simulink model "ProyectoAutomatasSimulink_jona2015a"  (R2015a)
settings: Solver=ode45  SolverMode=SingleTasking  StartTime=0.0  StopTime=100  RelTol=1e-3
undefined symbols (not defined in the file or in its folder): bh, bt, bw, g, Jh, Kw, Mh, ml, ml0, mlempty, mlfull, Mt, rc, Rd, rh, Rw, Thmax, Ttmax, yt0
settings Model: Creator=Maxi Garcia  LastModifiedBy=yellow submarine
settings DataIOCC: SignalLoggingSaveFormat=ModelDataLogs
settings OptimizationCC: BlockReduction=off  BooleanDataType=off
settings DebuggingCC: SaveWithParameterizedLinksMsg=none  UnderspecifiedInitializationDetection=Classic  MergeDetectMultiDrivingBlocksExec=none  SignalResolutionControl=TryResolveAllWithWarning  MultiTaskDSMMsg=warning  MultiTaskCondExecSysMsg=none
settings HardwareCC: TargetUnknown=on

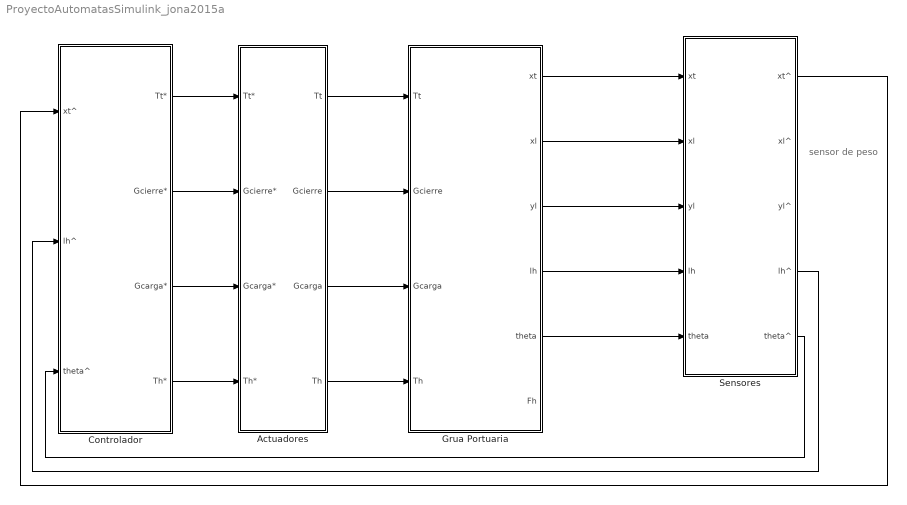
== system ProyectoAutomatasSimulink_jona2015a ==
  note: sensor de peso
  Actuadores : Subsystem
  Controlador : Subsystem
  Grua Portuaria : Subsystem
  Sensores : Subsystem
  wires:
  Grua Portuaria/1(xt) -> Sensores/1(xt)
  Grua Portuaria/2(xl) -> Sensores/2(xl)
  Grua Portuaria/3(yl) -> Sensores/3(yl)
  Grua Portuaria/4(lh) -> Sensores/4(lh)
  Grua Portuaria/5(theta) -> Sensores/5(theta)
  Actuadores/1(Tt) -> Grua Portuaria/1(Tt)
  Actuadores/2(Gcierre) -> Grua Portuaria/2(Gcierre)
  Actuadores/3(Gcarga) -> Grua Portuaria/3(Gcarga)
  Actuadores/4(Th) -> Grua Portuaria/4(Th)
  Controlador/1(Tt*) -> Actuadores/1(Tt*)
  Controlador/4(Th*) -> Actuadores/4(Th*)
  Controlador/2(Gcierre*) -> Actuadores/2(Gcierre*)
  Controlador/3(Gcarga*) -> Actuadores/3(Gcarga*)
  Sensores/5(theta^) -> Controlador/3(theta^)
  Sensores/4(lh^) -> Controlador/2(lh^)
  Sensores/1(xt^) -> Controlador/1(xt^)

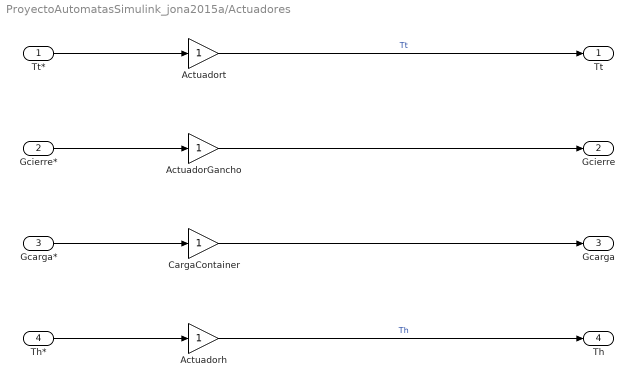
== system ProyectoAutomatasSimulink_jona2015a/Actuadores ==
  Tt* : Inport
  Gcierre* : Inport  Port=2
  Gcarga* : Inport  Port=3
  Th* : Inport  Port=4
  ActuadorGancho : Gain
  Actuadorh : Gain
  Actuadort : Gain
  CargaContainer : Gain
  Tt : Outport
  Gcierre : Outport  Port=2
  Gcarga : Outport  Port=3
  Th : Outport  Port=4
  wires:
  Th*/1 -> Actuadorh/1
  Actuadort/1 -> Tt/1  "Tt"
  Tt*/1 -> Actuadort/1
  ActuadorGancho/1 -> Gcierre/1
  CargaContainer/1 -> Gcarga/1
  Actuadorh/1 -> Th/1  "Th"
  Gcierre*/1 -> ActuadorGancho/1
  Gcarga*/1 -> CargaContainer/1

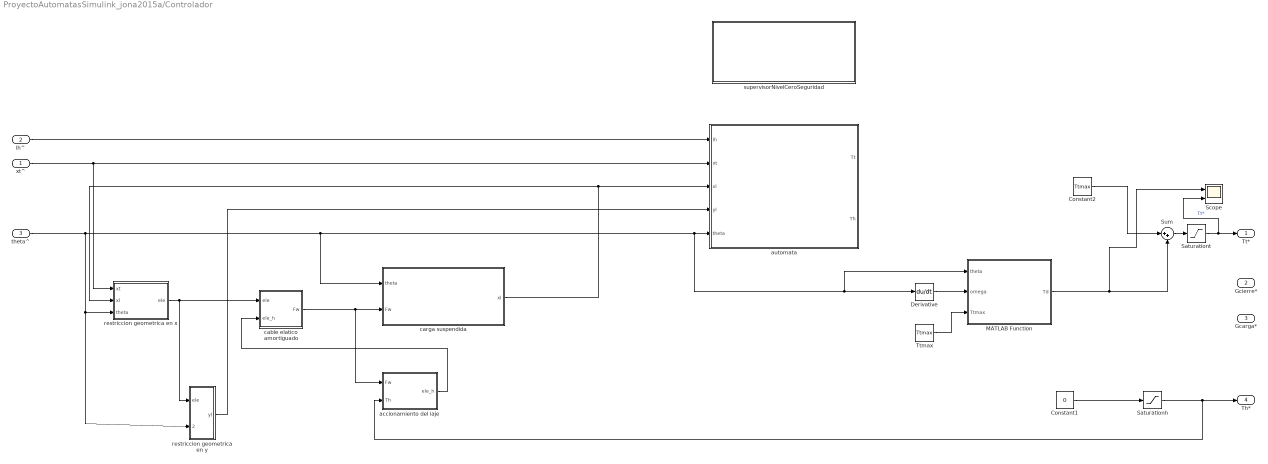
== system ProyectoAutomatasSimulink_jona2015a/Controlador ==
  xt^ : Inport
  lh^ : Inport  Port=2
  theta^ : Inport  Port=3
  Constant1 : Constant  Value=0
  Constant2 : Constant  Value=Ttmax
  Derivative : Derivative
  MATLAB Function : MATLAB Function  TreatAsAtomicUnit=on
      settings: PermitHierarchicalResolution=ParametersOnly
  Saturationh : Saturate  UpperLimit=Thmax  LowerLimit=-Ttmax
  Saturationt : Saturate  UpperLimit=Ttmax  LowerLimit=-Ttmax
  Scope : Scope  NumInputPorts=2
      settings: TimeRange=auto  MaxDataPoints=5000  SaveToWorkspace=off  YMin=-600000~-400000  YMax=800000~400000  SampleTime=-1  DataFormat=Array
  Sum : Sum  Inputs=|++
  Ttmax : Constant  Value=Ttmax
  accionamiento del iaje : Subsystem
  automata : Stateflow chart  TreatAsAtomicUnit=on
      settings: PermitHierarchicalResolution=ParametersOnly
  cable elatico amortiguado : Subsystem
  carga suspendida : Subsystem
  restriccion geometrica en x : Subsystem
  restriccion geometrica en y : Subsystem
  supervisorNivelCeroSeguridad : Stateflow chart  TreatAsAtomicUnit=on
      settings: PermitHierarchicalResolution=ParametersOnly
  Tt* : Outport
  Gcierre* : Outport  Port=2
  Gcarga* : Outport  Port=3
  Th* : Outport  Port=4
  wires:
  Saturationt/1 -> Scope/2, Tt*/1  "Tt*"
  MATLAB Function/1(Td) -> Sum/2, Scope/1
  Constant1/1 -> Saturationh/1
  theta^/1 -> restriccion geometrica en y/2(theta), restriccion geometrica en x/3(theta), carga suspendida/1(theta), Derivative/1, MATLAB Function/1(theta), automata/5(theta)
  Derivative/1 -> MATLAB Function/2(omega)
  Ttmax/1 -> MATLAB Function/3(Ttmax)
  Sum/1 -> Saturationt/1
  Constant2/1 -> Sum/1
  xt^/1 -> restriccion geometrica en x/1(xt), automata/2(xt)
  lh^/1 -> automata/1(lh)
  carga suspendida/1(xl) -> restriccion geometrica en x/2(xl), automata/3(xl)
  cable elatico amortiguado/1(Fw) -> accionamiento del iaje/1(Fw), carga suspendida/2(Fw)
  restriccion geometrica en x/1(ele) -> restriccion geometrica en y/1(ele), cable elatico amortiguado/1(ele)
  Saturationh/1 -> accionamiento del iaje/2(Th), Th*/1
  accionamiento del iaje/1(ele_h) -> cable elatico amortiguado/2(ele_h)
  restriccion geometrica en y/1(yl) -> automata/4(yl)

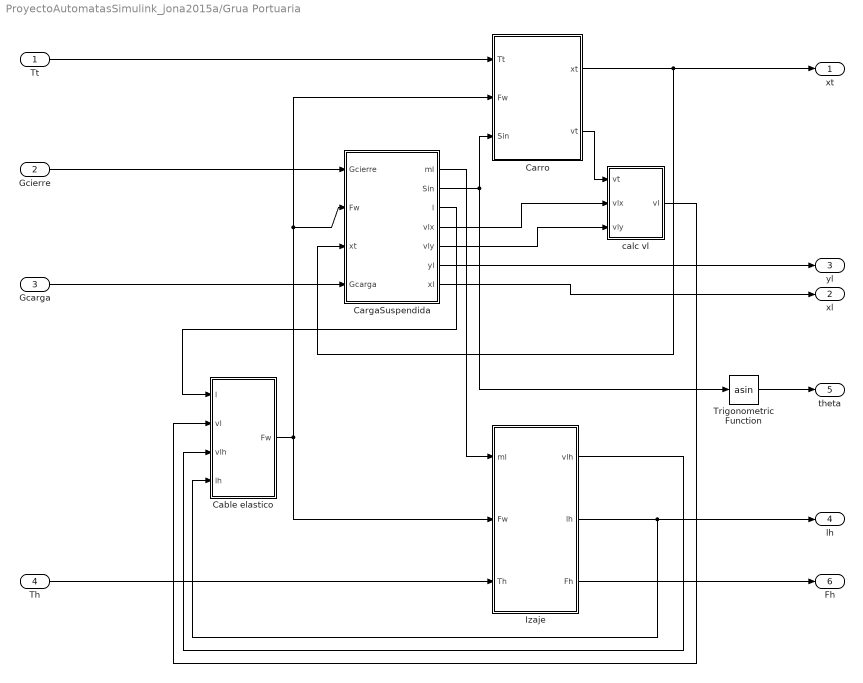
== system ProyectoAutomatasSimulink_jona2015a/Grua Portuaria ==
  Tt : Inport
  Gcierre : Inport  Port=2
  Gcarga : Inport  Port=3
  Th : Inport  Port=4
  Cable elastico : Subsystem
  CargaSuspendida : Subsystem
  Carro : Subsystem
  Izaje : Subsystem
  Trigonometric Function : Trigonometry  Operator=asin
  calc vl : Subsystem
  xt : Outport
  xl : Outport  Port=2
  yl : Outport  Port=3
  lh : Outport  Port=4
  theta : Outport  Port=5
  Fh : Outport  Port=6
  wires:
  Izaje/1(vlh) -> Cable elastico/3(vlh)
  CargaSuspendida/2(Sin) -> Carro/3(Sin), Trigonometric Function/1
  Th/1 -> Izaje/3(Th)
  Izaje/2(lh) -> Cable elastico/4(lh), lh/1
  Carro/1(xt) -> xt/1, CargaSuspendida/3(xt)
  CargaSuspendida/1(ml) -> Izaje/1(ml)
  Gcierre/1 -> CargaSuspendida/1(Gcierre)
  Gcarga/1 -> CargaSuspendida/4(Gcarga)
  Tt/1 -> Carro/1(Tt)
  CargaSuspendida/3(l) -> Cable elastico/1(l)
  Carro/2(vt) -> calc vl/1(vt)
  CargaSuspendida/4(vlx) -> calc vl/2(vlx)
  CargaSuspendida/5(vly) -> calc vl/3(vly)
  calc vl/1(vl) -> Cable elastico/2(vl)
  Cable elastico/1(Fw) -> Izaje/2(Fw), CargaSuspendida/2(Fw), Carro/2(Fw)
  CargaSuspendida/6(yl) -> yl/1
  CargaSuspendida/7(xl) -> xl/1
  Trigonometric Function/1 -> theta/1
  Izaje/3(Fh) -> Fh/1

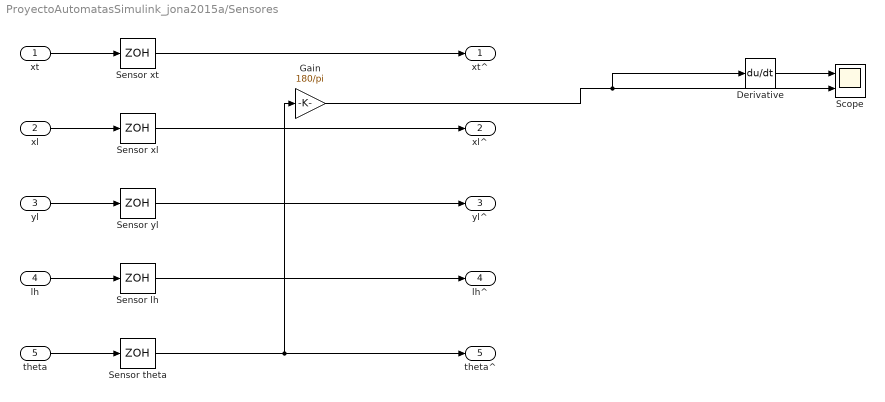
== system ProyectoAutomatasSimulink_jona2015a/Sensores ==
  xt : Inport
  xl : Inport  Port=2
  yl : Inport  Port=3
  lh : Inport  Port=4
  theta : Inport  Port=5
  Derivative : Derivative
  Gain : Gain  Gain=180/pi
  Scope : Scope  NumInputPorts=2
      settings: TimeRange=auto  MaxDataPoints=5000  SaveToWorkspace=off  SaveName=ScopeData  YMin=0~-2.25  YMax=7500~0.5  SampleTime=-1  DataFormat=Array
  Sensor lh : ZeroOrderHold  SampleTime=0.01
  Sensor theta : ZeroOrderHold  SampleTime=0.01
  Sensor xl : ZeroOrderHold  SampleTime=0.01
  Sensor xt : ZeroOrderHold  SampleTime=0.01
  Sensor yl : ZeroOrderHold  SampleTime=0.01
  xt^ : Outport
  xl^ : Outport  Port=2
  yl^ : Outport  Port=3
  lh^ : Outport  Port=4
  theta^ : Outport  Port=5
  wires:
  xt/1 -> Sensor xt/1
  theta/1 -> Sensor theta/1
  xl/1 -> Sensor xl/1
  yl/1 -> Sensor yl/1
  Sensor lh/1 -> lh^/1
  Sensor yl/1 -> yl^/1
  Sensor xl/1 -> xl^/1
  Sensor xt/1 -> xt^/1
  Sensor theta/1 -> Gain/1, theta^/1
  lh/1 -> Sensor lh/1
  Gain/1 -> Derivative/1, Scope/2
  Derivative/1 -> Scope/1

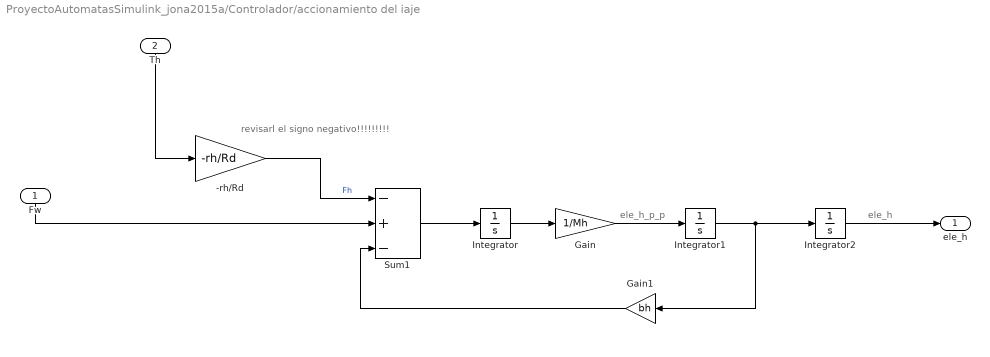
== system ProyectoAutomatasSimulink_jona2015a/Controlador/accionamiento del iaje ==
  note: revisarl el signo negativo!!!!!!!!!
  note: ele_h
  note: ele_h_p_p
  Fw : Inport
  Th : Inport  Port=2
  "-rh/Rd\t" : Gain  Gain=-rh/Rd
  Gain : Gain  Gain=1/Mh
  Gain1 : Gain  Gain=bh
  Integrator : Integrator
  Integrator1 : Integrator
  Integrator2 : Integrator
  Sum1 : Sum  Inputs=-+-
  ele_h : Outport
  wires:
  Integrator1/1 -> Gain1/1, Integrator2/1
  Sum1/1 -> Integrator/1
  Gain/1 -> Integrator1/1
  "-rh/Rd\t"/1 -> Sum1/1  "Fh"
  Integrator/1 -> Gain/1
  Th/1 -> "-rh/Rd\t"/1
  Fw/1 -> Sum1/2
  Gain1/1 -> Sum1/3
  Integrator2/1 -> ele_h/1

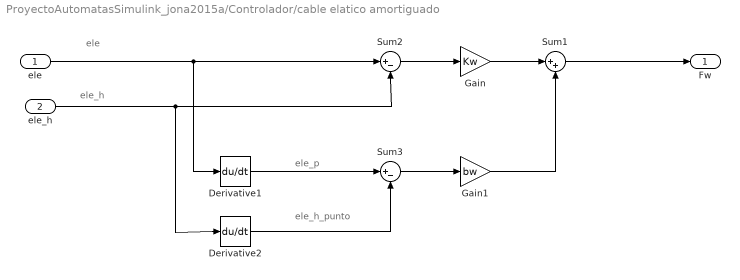
== system ProyectoAutomatasSimulink_jona2015a/Controlador/cable elatico amortiguado ==
  note: ele_h_punto
  note: ele_p
  note: ele_h
  note: ele
  ele : Inport
  ele_h : Inport  Port=2
  Derivative1 : Derivative
  Derivative2 : Derivative
  Gain : Gain  Gain=Kw
  Gain1 : Gain  Gain=bw
  Sum1 : Sum  Inputs=|++
  Sum2 : Sum  Inputs=|+-
  Sum3 : Sum  Inputs=|+-
  Fw : Outport
  wires:
  ele_h/1 -> Derivative2/1, Sum2/2
  Sum2/1 -> Gain/1
  Sum3/1 -> Gain1/1
  ele/1 -> Derivative1/1, Sum2/1
  Derivative1/1 -> Sum3/1
  Gain1/1 -> Sum1/2
  Gain/1 -> Sum1/1
  Sum1/1 -> Fw/1
  Derivative2/1 -> Sum3/2

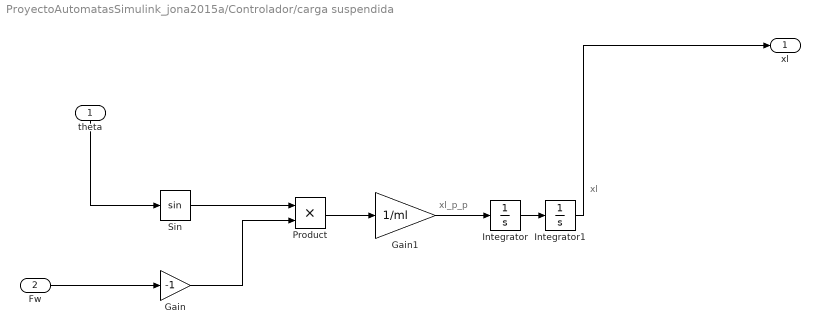
== system ProyectoAutomatasSimulink_jona2015a/Controlador/carga suspendida ==
  note: xl
  note: xl_p_p
  theta : Inport
  Fw : Inport  Port=2
  Gain : Gain  Gain=-1
  Gain1 : Gain  Gain=1/ml
  Integrator : Integrator
  Integrator1 : Integrator
  Product : Product
  Sin : Trigonometry
  xl : Outport
  wires:
  Integrator1/1 -> xl/1
  theta/1 -> Sin/1
  Sin/1 -> Product/1
  Gain1/1 -> Integrator/1
  Product/1 -> Gain1/1
  Integrator/1 -> Integrator1/1
  Fw/1 -> Gain/1
  Gain/1 -> Product/2

== system ProyectoAutomatasSimulink_jona2015a/Controlador/restriccion geometrica en x ==
  xt : Inport
  xl : Inport  Port=2
  theta : Inport  Port=3
  Divide : Product  Inputs=*/
  Sin : Trigonometry
  Sum1 : Sum  Inputs=|+-
  ele : Outport
  wires:
  Divide/1 -> ele/1
  Sum1/1 -> Divide/1
  Sin/1 -> Divide/2
  xl/1 -> Sum1/1
  theta/1 -> Sin/1
  xt/1 -> Sum1/2

== system ProyectoAutomatasSimulink_jona2015a/Controlador/restriccion geometrica en y ==
  note: yl
  ele : Inport
  theta : Inport  Port=2
  Constant : Constant  Value=yt0
  Cos : Trigonometry  Operator=cos
  Product : Product
  Sum1 : Sum  Inputs=|+-
  yl : Outport
  wires:
  theta/1 -> Cos/1
  ele/1 -> Product/1
  Sum1/1 -> yl/1
  Product/1 -> Sum1/2
  Constant/1 -> Sum1/1
  Cos/1 -> Product/2

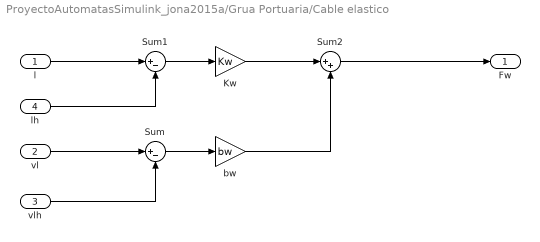
== system ProyectoAutomatasSimulink_jona2015a/Grua Portuaria/Cable elastico ==
  l : Inport
  vl : Inport  Port=2
  vlh : Inport  Port=3
  lh : Inport  Port=4
  Kw : Gain  Gain=Kw
  Sum : Sum  Inputs=|+-
  Sum1 : Sum  Inputs=|+-
  Sum2 : Sum  Inputs=|++
  bw : Gain  Gain=bw
  Fw : Outport
  wires:
  l/1 -> Sum1/1
  lh/1 -> Sum1/2
  vl/1 -> Sum/1
  vlh/1 -> Sum/2
  Sum1/1 -> Kw/1
  Sum2/1 -> Fw/1
  Sum/1 -> bw/1
  Kw/1 -> Sum2/1
  bw/1 -> Sum2/2

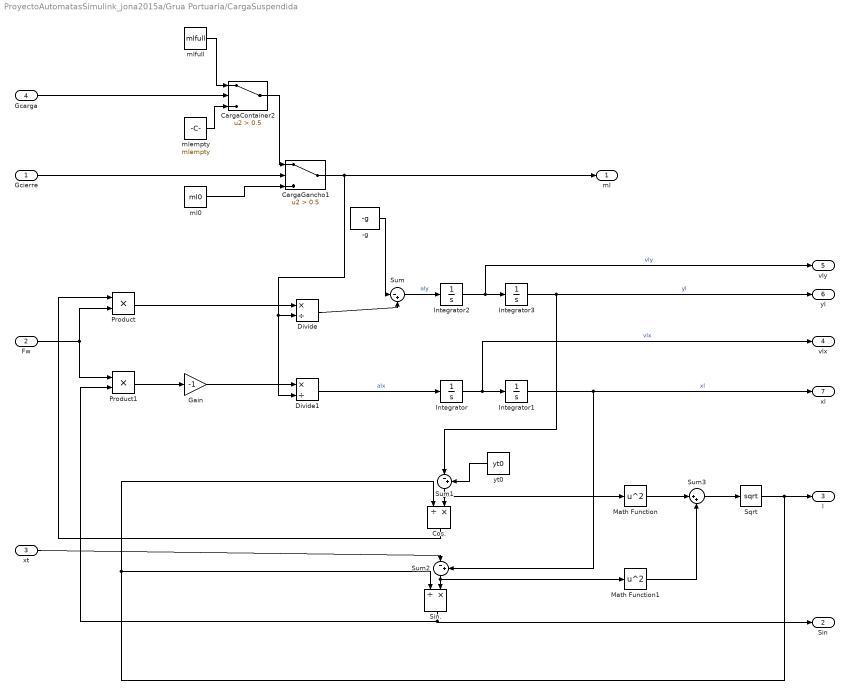
== system ProyectoAutomatasSimulink_jona2015a/Grua Portuaria/CargaSuspendida ==
  Gcierre : Inport
  Fw : Inport  Port=2
  xt : Inport  Port=3
  Gcarga : Inport  Port=4
  -g : Constant  Value=-g
  CargaContainer2 : Switch  Criteria=u2 > Threshold  Threshold=0.5
  CargaGancho1 : Switch  Criteria=u2 > Threshold  Threshold=0.5
  Cos. : Product  Inputs=/*
  Divide : Product  Inputs=*/
  Divide1 : Product  Inputs=*/
  Gain : Gain  Gain=-1
  Integrator{,1..3} (4 alike) : Integrator
  Math Function : Math  Operator=square  SaturateOnIntegerOverflow=on
  Math Function1 : Math  Operator=square  SaturateOnIntegerOverflow=on
  Product : Product
  Product1 : Product
  Sin. : Product  Inputs=/*
  Sqrt : Sqrt  SaturateOnIntegerOverflow=on
  Sum : Sum  Inputs=|-+
  Sum1 : Sum  Inputs=|-+
  Sum2 : Sum  Inputs=|-+
  Sum3 : Sum  Inputs=|++
  "ml0 " : Constant  Value=ml0
  mlempty : Constant  Value=mlempty
  mlfull : Constant  Value=mlfull
  yt0 : Constant  Value=yt0
  ml : Outport
  Sin : Outport  Port=2
  l : Outport  Port=3
  vlx : Outport  Port=4
  vly : Outport  Port=5
  yl : Outport  Port=6
  xl : Outport  Port=7
  wires:
  CargaGancho1/1 -> Divide/2, Divide1/2, ml/1
  Gcierre/1 -> CargaGancho1/2
  Sqrt/1 -> Cos./1, Sin./1, l/1
  Fw/1 -> Product1/1, Product/2
  Product/1 -> Divide/1
  Product1/1 -> Gain/1
  Gain/1 -> Divide1/1
  Divide/1 -> Sum/2
  -g/1 -> Sum/1
  Divide1/1 -> Integrator/1  "alx"
  Integrator/1 -> vlx/1, Integrator1/1  "vlx"
  Integrator1/1 -> xl/1, Sum2/2  "xl"
  Integrator2/1 -> vly/1, Integrator3/1  "vly"
  Sum/1 -> Integrator2/1  "aly"
  Sum1/1 -> Cos./2, Math Function/1
  yt0/1 -> Sum1/2
  Integrator3/1 -> Sum1/1, yl/1  "yl"
  Cos./1 -> Product/1
  Sum2/1 -> Math Function1/1, Sin./2
  xt/1 -> Sum2/1
  Sin./1 -> Sin/1, Product1/2
  Math Function/1 -> Sum3/1
  Math Function1/1 -> Sum3/2
  Sum3/1 -> Sqrt/1
  CargaContainer2/1 -> CargaGancho1/1
  Gcarga/1 -> CargaContainer2/2
  "ml0 "/1 -> CargaGancho1/3
  mlempty/1 -> CargaContainer2/3
  mlfull/1 -> CargaContainer2/1

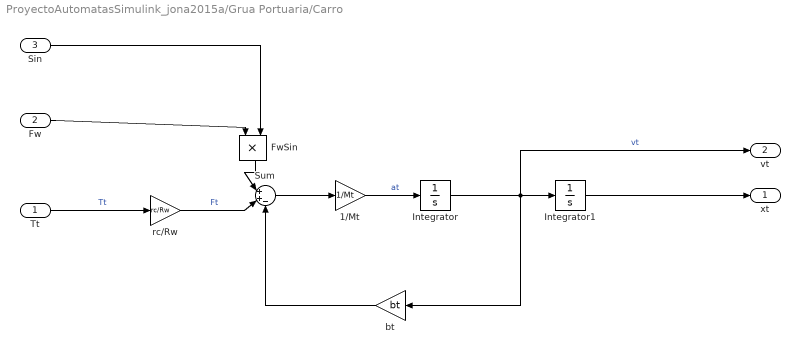
== system ProyectoAutomatasSimulink_jona2015a/Grua Portuaria/Carro ==
  Tt : Inport
  Fw : Inport  Port=2
  Sin : Inport  Port=3
  1/Mt : Gain  Gain=1/Mt
  FwSin : Product
  Integrator : Integrator
  Integrator1 : Integrator
  Sum : Sum  Inputs=|++-
  bt : Gain  Gain=bt
  rc/Rw : Gain  Gain=rc/Rw
  xt : Outport
  vt : Outport  Port=2
  wires:
  Integrator1/1 -> xt/1
  rc/Rw/1 -> Sum/2  "Ft"
  Tt/1 -> rc/Rw/1  "Tt"
  1/Mt/1 -> Integrator/1  "at"
  bt/1 -> Sum/3
  Sum/1 -> 1/Mt/1
  Integrator/1 -> bt/1, vt/1, Integrator1/1  "vt"
  Sin/1 -> FwSin/2
  FwSin/1 -> Sum/1
  Fw/1 -> FwSin/1

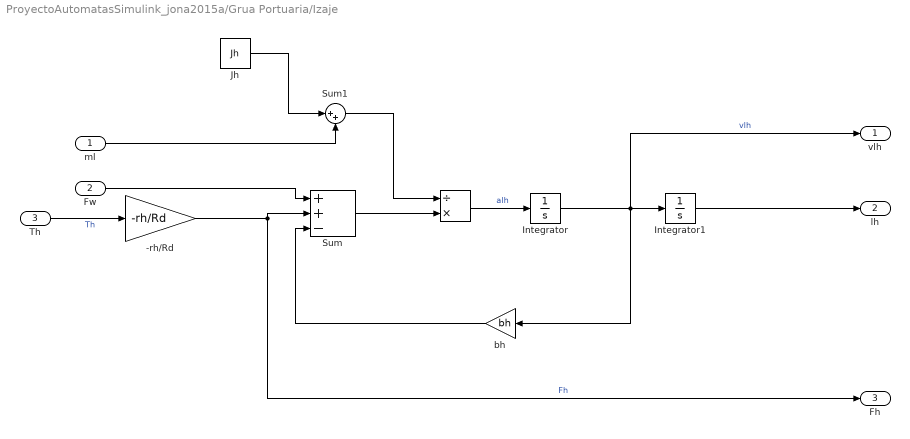
== system ProyectoAutomatasSimulink_jona2015a/Grua Portuaria/Izaje ==
  ml : Inport
  Fw : Inport  Port=2
  Th : Inport  Port=3
  " " : Product  Inputs=/*
  "-rh/Rd\t" : Gain  Gain=-rh/Rd
  Integrator : Integrator
  Integrator1 : Integrator
  Jh : Constant  Value=Jh
  Sum : Sum  Inputs=|++-
  Sum1 : Sum  Inputs=|++
  bh : Gain  Gain=bh
  vlh : Outport
  lh : Outport  Port=2
  Fh : Outport  Port=3
  wires:
  Integrator1/1 -> lh/1
  "-rh/Rd\t"/1 -> Fh/1, Sum/2  "Fh"
  Th/1 -> "-rh/Rd\t"/1  "Th"
  " "/1 -> Integrator/1  "alh"
  bh/1 -> Sum/3
  Sum/1 -> " "/2
  Integrator/1 -> vlh/1, bh/1, Integrator1/1  "vlh"
  Fw/1 -> Sum/1
  ml/1 -> Sum1/2
  Sum1/1 -> " "/1
  Jh/1 -> Sum1/1

== system ProyectoAutomatasSimulink_jona2015a/Grua Portuaria/calc vl ==
  vt : Inport
  vlx : Inport  Port=2
  vly : Inport  Port=3
  Math Function : Math  Operator=square  SaturateOnIntegerOverflow=on
  Math Function1 : Math  Operator=square  SaturateOnIntegerOverflow=on
  Sqrt : Sqrt  SaturateOnIntegerOverflow=on
  Sum1 : Sum  Inputs=|+-
  Sum3 : Sum  Inputs=|++
  vl : Outport
  wires:
  Sqrt/1 -> vl/1
  Math Function1/1 -> Sum3/2
  Math Function/1 -> Sum3/1
  Sum3/1 -> Sqrt/1
  vly/1 -> Math Function/1
  vlx/1 -> Sum1/1
  Sum1/1 -> Math Function1/1
  vt/1 -> Sum1/2

== stateflow chart ProyectoAutomatasSimulink_jona2015a/Controlador/supervisorNivelCeroSeguridad ==

== matlab function ProyectoAutomatasSimulink_jona2015a/Controlador/MATLAB Function ==
  data: theta input; Td output; omega input; Ttmax input
function Td = LogicaDifusa(theta,omega,Ttmax)
%#codegen
rad = 180/pi;
theta=theta*rad;
omega=omega*rad;
Reglas=[-1,-1,-0.5,-0.5,0
-1,-0.5,-0.5,0,0.5
-0.5,-0.5,0,0.5,0.5
-0.5,0,0.5,0.5,1
0,0.5,0.5,1,1];
Reglas=Reglas*Ttmax;
PertTita=[0,0,0,0,0];
Pertw=[0,0,0,0,0];
CentrosPonderados=0;
CentrosDenominador=0;
if(theta<=-30)
   PertTita(1)=1;
end
if(theta>-30 && theta<=-15)
   PertTita(1)=-(theta+15)/15;
   PertTita(2)=1+(theta+15)/15;
end
if(theta>=-15 && theta<0)
   PertTita(2)=-theta/15;
   PertTita(3)=1+theta/15;
end
if(theta>=0 && theta<15)
   PertTita(3)=-(theta-15)/15;
   PertTita(4)=1+(theta-15)/15;
end
if(theta>=15 && theta<30)
   PertTita(4)=-(theta-30)/15;
   PertTita(5)=1+(theta-30)/15;
end
if(theta>=30)
   PertTita(5)=1;
end
if(omega<=-30)
   Pertw(1)=1;
end
if(omega>-30 && omega<=-15)
   Pertw(1)=-(omega+15)/15;
   Pertw(2)=1+(omega+15)/15;
end
if(omega>=-15 && omega<0)
   Pertw(2)=-omega/15;
   Pertw(3)=1+omega/15;
end
if(omega>=0 && omega<15)
   Pertw(3)=-(omega-15)/15;
   Pertw(4)=1+(omega-15)/15;
end
if(omega>=15 && omega<30)
   Pertw(4)=-(omega-30)/15;
   Pertw(5)=1+(omega-30)/15;
end
if(omega>=30)
   Pertw(5)=1;
end
for i=1:5
        for j=1:5
            if(Pertw(i)<PertTita(j))
                CentrosPonderados=CentrosPonderados+Reglas(i,j)*Pertw(i);
                CentrosDenominador=CentrosDenominador+Pertw(i);
            else
                CentrosPonderados=CentrosPonderados+Reglas(i,j)*PertTita(j);
                CentrosDenominador=CentrosDenominador+PertTita(j);
            end
        end
end

Fuerza=CentrosPonderados/CentrosDenominador;
Td = Fuerza;

== stateflow chart ProyectoAutomatasSimulink_jona2015a/Controlador/automata ==
  state inicio
  state maquinaOperando
    state verificaLimites [parallel]
      settings: executionOrder=2
      state ganchoLimiteMaximo
      state dentroDeLimites
      state carroLimiteMinimo
      state ganchoLimiteMinimo
      state carroLimiteMaximo
      (default) -> dentroDeLimites
      dentroDeLimites -> carroLimiteMinimo [order 1] : [xt<=xt_min]
      ganchoLimiteMaximo -> dentroDeLimites : [l<=l_max_cable]
      dentroDeLimites -> ganchoLimiteMaximo [order 3] : [l>=l_max_cable]
      carroLimiteMinimo -> dentroDeLimites : [xt>xt_min]
      dentroDeLimites -> carroLimiteMaximo [order 2] : [xt>=xt_max]
      carroLimiteMaximo -> dentroDeLimites : [xt<xt_max]
      ganchoLimiteMinimo -> dentroDeLimites : [l<=l_min_cable]
      dentroDeLimites -> ganchoLimiteMinimo [order 4] : [l>=l_min_cable]
    state modoDeOperacion [parallel]
      settings: executionOrder=3
      state opManual
      state opAutomatica
      state transfiriendoModo
      (default) -> opManual
      opAutomatica -> opManual : {modoAutomatico=0}
      opManual -> transfiriendoModo : {modoAutomatico=1}
      transfiriendoModo -> opAutomatica : {modoAutomatico=1}
    state gancho [parallel]
      settings: executionOrder=1
      state Gabierto
      state Gcerrado
      (default) -> Gabierto
      Gcerrado -> Gabierto : {cerrarGancho=0}
      Gabierto -> Gcerrado : {cerrarGancho=1}
  state configuracion
  (default) -> inicio
  maquinaOperando -> inicio : {operar_maq=0}
  inicio -> maquinaOperando [order 2] : {operar_maq=1}
  inicio -> configuracion [order 1] : {aprendizaje=1}
  configuracion -> inicio : {aprendizaje=0}
  data: lh input; lx_max constant double; xt input; xl input; yl input; theta input; Tt output; Th output
